simulink model "torque11"  (Simulink 8.9)
settings: Solver=ode5  StartTime=0.0  StopTime=2.7625  FixedStep=0.005  RelTol=1e-3  AbsTol=1e-6  EnableMultiTasking=on
values from neighbouring files (symbols this model uses):
  Kp = 6*a.*omega.^2    [init_PID.m]    (also in init_torque.m = omega.^2)
  kt = [20 7]    [init_PID.m]    (also in init_torque.m)
  Kv = 2*chi*omega    [init_torque.m]
  ListePoints = [100*pi/360 100*pi/360;6*pi/360 60*pi/360]    [init_PID.m]    (also in init_torque.m)
undefined symbols (not defined in the file or in its folder): inter_arti_d5, scarabase_ddm, scarabase_dyn
settings Model: SuppressorTable=22 serialization::archive 11 0 6 0 0 0 11 0  Creator=user  LastModifiedBy=steff  ExtModeTrigMode=oneshot  ExtModeArmWhenConnect=off
settings DataIOCC: LimitDataPoints=off  SignalLoggingName=sigsOut
settings OptimizationCC: BooleanDataType=off  ExpressionDepthLimit=2147483647
settings DebuggingCC: SaveWithParameterizedLinksMsg=none  SignalResolutionControl=TryResolveAllWithWarning  MultiTaskDSMMsg=warning  MultiTaskCondExecSysMsg=none  FcnCallInpInsideContextMsg=error
settings HardwareCC: TargetUnknown=on
settings RTWCC: TemplateMakefile=grt_vc.tmf

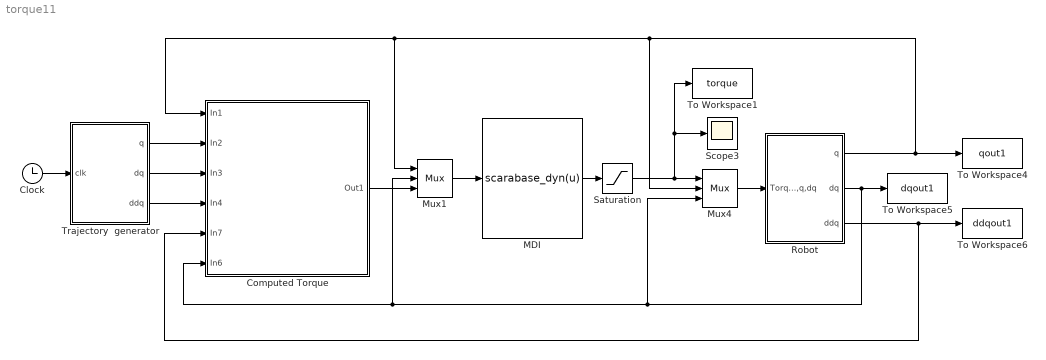
== system torque11 ==
  Clock : Clock
  Computed Torque : Subsystem
  MDI : MATLABFcn  MATLABFcn=scarabase_dyn(u)  OutputDimensions=2  Output1D=off
  Mux1 : Mux  Inputs=3
  Mux4 : Mux  Inputs=3
  Robot : Subsystem
  Saturation : Saturate  UpperLimit=kt  LowerLimit=-kt
  Scope3 : Scope
  To Workspace1 : ToWorkspace  VariableName=torque  SampleTime=-1
  To Workspace4 : ToWorkspace  VariableName=qout1  SampleTime=-1
  To Workspace5 : ToWorkspace  VariableName=dqout1  SampleTime=-1
  To Workspace6 : ToWorkspace  VariableName=ddqout1  SampleTime=-1
  Trajectory  generator : Subsystem
  wires:
  MDI/1 -> Saturation/1
  Mux1/1 -> MDI/1
  Saturation/1 -> To Workspace1/1, Scope3/1, Mux4/1
  Clock/1 -> Trajectory  generator/1(clk)
  Robot/3(ddq) -> Computed Torque/5(In7), To Workspace6/1
  Robot/2(dq) -> To Workspace5/1, Mux4/3, Computed Torque/6(In6), Mux1/2
  Mux4/1 -> Robot/1(Torque,q,dq)
  Robot/1(q) -> To Workspace4/1, Mux4/2, Mux1/1, Computed Torque/1(In1)
  Trajectory  generator/1(q) -> Computed Torque/2(In2)
  Trajectory  generator/2(dq) -> Computed Torque/3(In3)
  Trajectory  generator/3(ddq) -> Computed Torque/4(In4)
  Computed Torque/1(Out1) -> Mux1/3

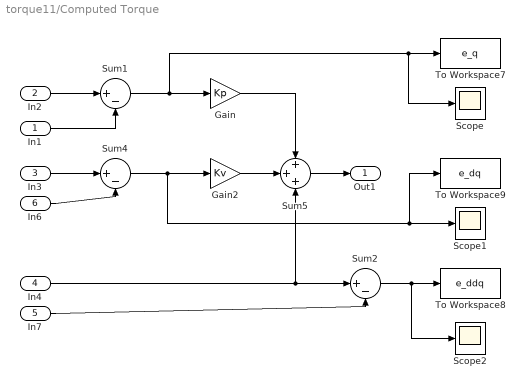
== system torque11/Computed Torque ==
  In1 : Inport
  In2 : Inport  Port=2
  In3 : Inport  Port=3
  In4 : Inport  Port=4
  In7 : Inport  Port=5
  In6 : Inport  Port=6
  Gain : Gain  Gain=Kp
  Gain2 : Gain  Gain=Kv
  Scope : Scope
  Scope1 : Scope
  Scope2 : Scope
  Sum1 : Sum  Inputs=|+-  SaturateOnIntegerOverflow=on
  Sum2 : Sum  Inputs=|+-  SaturateOnIntegerOverflow=on
  Sum4 : Sum  Inputs=|+-  SaturateOnIntegerOverflow=on
  Sum5 : Sum  Inputs=+++
  To Workspace7 : ToWorkspace  VariableName=e_q  SampleTime=-1
  To Workspace8 : ToWorkspace  VariableName=e_ddq  SampleTime=-1
  To Workspace9 : ToWorkspace  VariableName=e_dq  SampleTime=-1
  Out1 : Outport
  wires:
  Sum4/1 -> To Workspace9/1, Scope1/1, Gain2/1
  Gain2/1 -> Sum5/2
  Sum2/1 -> Scope2/1, To Workspace8/1
  Sum1/1 -> To Workspace7/1, Scope/1, Gain/1
  Gain/1 -> Sum5/1
  In4/1 -> Sum5/3, Sum2/1
  Sum5/1 -> Out1/1
  In3/1 -> Sum4/1
  In6/1 -> Sum4/2
  In2/1 -> Sum1/1
  In1/1 -> Sum1/2
  In7/1 -> Sum2/2

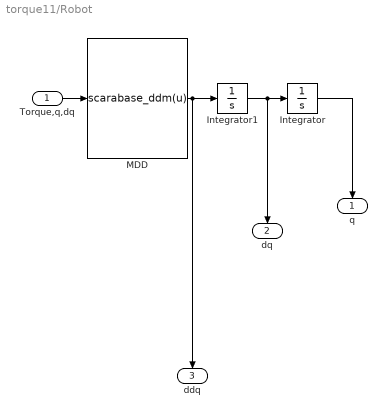
== system torque11/Robot ==
  Torque,q,dq : Inport
  Integrator : Integrator  InitialCondition=ListePoints(1,:)
  Integrator1 : Integrator  InitialCondition=[0 0]
  MDD : MATLABFcn  MATLABFcn=scarabase_ddm(u)  OutputDimensions=2
  q : Outport
  dq : Outport  Port=2
  ddq : Outport  Port=3
  wires:
  Integrator1/1 -> dq/1, Integrator/1
  Integrator/1 -> q/1
  MDD/1 -> ddq/1, Integrator1/1
  Torque,q,dq/1 -> MDD/1

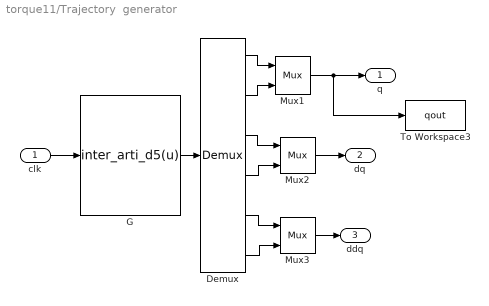
== system torque11/Trajectory  generator ==
  clk : Inport
  Demux : Demux  Outputs=6
  G : MATLABFcn  MATLABFcn=inter_arti_d5(u)  OutputDimensions=6  Output1D=off
  Mux1 : Mux  Inputs=2
  Mux2 : Mux  Inputs=2
  Mux3 : Mux  Inputs=2
  To Workspace3 : ToWorkspace  VariableName=qout  SampleTime=-1
  q : Outport
  dq : Outport  Port=2
  ddq : Outport  Port=3
  wires:
  Demux/1 -> Mux1/1
  Demux/6 -> Mux3/2
  Demux/3 -> Mux2/1
  Mux2/1 -> dq/1
  Demux/2 -> Mux1/2
  Demux/4 -> Mux2/2
  Demux/5 -> Mux3/1
  clk/1 -> G/1
  Mux3/1 -> ddq/1
  G/1 -> Demux/1
  Mux1/1 -> To Workspace3/1, q/1
